simulink model "Sim_Multi"  (R2016b)
settings: Solver=ode3  StartTime=0.0  StopTime=sim_time  FixedStep=t_sim  MaxStep=t_control  RelTol=1e-5  EnableMultiTasking=on
values from neighbouring files (symbols this model uses):
  Att_init = [0;0;0] * d2r    [Init_Multi.m]
  Blade_flapping = 0    [Init_Multi.m]
  C_D = 0.40    (= 0.4)    [Init_Multi.m]
  CoG_nominal = [0;0;0.001]    [Init_Multi.m]
  CoG_real = [0;0;0.001]    [Init_Multi.m]
  Coriolis_correction = 1    [Init_Multi.m]
  d2r = pi/180    (= 0.0174532925199)    [Init_Multi.m]
  Dyn_thrust = 0    [Init_Multi.m]
  g = 9.80665    [Init_Multi.m]
  J_nominal = [Jxx Jxy Jxz;Jyx Jyy Jyz;Jzx Jzy Jzz]    [Init_Multi.m]
  J_real = [Jxx Jxy Jxz;Jyx Jyy Jyz;Jzx Jzy Jzz]    [Init_Multi.m]
  k1 = -1.125    [Init_Multi.m]
  k2 = -1.372    [Init_Multi.m]
  k3 = -1.718    [Init_Multi.m]
  k4 = -0.655    [Init_Multi.m]
  k_a1s = 1.5 / 4.0    (= 0.375)    [Init_Multi.m]
  k_beta = 0.23    [Init_Multi.m]
  kappa = 1.00    (= 1)    [Init_Multi.m]
  Kff_1 = 0.7*[1;1;0.95]    [Init_Multi.m]
  Ki_1 = 10*[1;1;1.5]    [Init_Multi.m]
  Kp_1 = 15*[1;1;1.5]    [Init_Multi.m]
  mass_nominal = 0.550    (= 0.55)    [Init_Multi.m]
  mass_real = 0.550    (= 0.55)    [Init_Multi.m]
  max_thrust = max_thrust + (MotorMatrix_nominal(i,7)*MotorMatrix_nominal(i,12)+MotorMatrix_nominal(i,8)*MotorMatrix_nominal(i,12)^2)    [Init_Multi.m]
  MaxRate_cmd = [360;360;120] * d2r    [Init_Multi.m]
  min_thrust = min_thrust + (MotorMatrix_nominal(i,7)*MotorMatrix_nominal(i,11)+MotorMatrix_nominal(i,8)*MotorMatrix_nominal(i,11)^2)    [Init_Multi.m]
  MotorMap = B' * inv(B * B')    [Init_Multi.m]
  MotorMatrix_nominal = [045 , 0.170 , -0.028 , -1 , 1.0 , 0.010 , [9.6820 , 0.010872]*1e-5 , [1.4504 , 0.0016312]*1e-6 , 0000 , 6000 , [0.0 , 0.0 , 0.0] , 8*2.54/100 , 11/1000;                         135 , 0.170 , -0.028 , +1 , 1.0 , 0.010 , [9.6820 , 0.010872]*1e-5 , [1.4504 , 0.0016312]*1e-6 , 0000 , 6000 , [0.0 , 0.0 , 0.0] , 8*2.54/100 , 11/1000;                         225 , 0.170 , -0.028 , -1 , 1.0 , 0.010 , [9. ...(+284 chars)    [Init_Multi.m]
  MotorMatrix_real = [045 , 0.170 , -0.028 , -1 , 1.0 , 0.010 , [9.6820 , 0.010872]*1e-5 , [1.4504 , 0.0016312]*1e-6 , 0000 , 6000 , [0.0 , 0.0 , 0.0] , 8*2.54/100 , 11/1000;                      135 , 0.170 , -0.028 , +1 , 1.0 , 0.010 , [9.6820 , 0.010872]*1e-5 , [1.4504 , 0.0016312]*1e-6 , 0000 , 6000 , [0.0 , 0.0 , 0.0] , 8*2.54/100 , 11/1000;                      225 , 0.170 , -0.028 , -1 , 1.0 , 0.010 , [9.6820 , ...(+275 chars)    [Init_Multi.m]
  Noise_flag = 0    [Init_Multi.m]
  omega_init = [0;0;0]    [Init_Multi.m]
  q_init = rpy2quat(Att_init)    [Init_Multi.m]
  r2d = 180/pi    (= 57.2957795131)    [Init_Multi.m]
  rho = 1.225    [Init_Multi.m]
  rpm2radpersec = 2*pi/60    (= 0.10471975512)    [Init_Multi.m]
  rpm_init = 3104.5025852    [Init_Multi.m]
  Surface_params = [a;b;c]    [Init_Multi.m]
  t_control = 1/500    (= 0.002)    [Init_Multi.m]
  t_sim = t_control/2    (= 0.001)    [Init_Multi.m]
  thrust_gain = (max_thrust - min_thrust) / 1000    (= 0)    [Init_Multi.m]
  thrust_offset = min_thrust    (= 0)    [Init_Multi.m]
  thrust_reserve = 0.10    (= 0.1)    [Init_Multi.m]
  v_h = 4.0    (= 4)    [Init_Multi.m]
  Vb_init = [0;0;0]    [Init_Multi.m]
  Vi_init = R_IB_init' * Vb_init    [Init_Multi.m]
  Xi_init = [0;0;0]    [Init_Multi.m]
undefined symbols (not defined in the file or in its folder): DiscIntNeverNeededParam, rpy2quat, thrust2rpm
libraries: simulink x17
(part 4 of 4)

== system Sim_Multi/True dynamic system representation of a multirotor UAV/Force//Moment computation/Forces and moments generated by spinning propellers/For Each Subsystem/Thrust//moment vector for each propeller (Body axes)/Compute dynamic motor thrust and moments/Dynamic thrust ratio/Angle of attack and airspeed magnitude/Nonzero airspeed ==
  Airspeed (Motor) : Inport
  Action Port : ActionPort  ActionType=else
  Demux : Demux  Outputs=[2,1]
  Divide1 : Product  Inputs=/*
  Trigonometric Function : Trigonometry  Operator=atan
  norm1 : Subsystem
  AoA (rad) : Outport
  wires:
  Trigonometric Function/1 -> AoA (rad)/1
  Demux/1 -> norm1/1(u)  "Airspeed xy component"
  Demux/2 -> Divide1/2  "Airspeed z component"
  norm1/1(||u||) -> Divide1/1
  Divide1/1 -> Trigonometric Function/1
  Airspeed (Motor)/1 -> Demux/1

== system Sim_Multi/True dynamic system representation of a multirotor UAV/Force//Moment computation/Forces and moments generated by spinning propellers/For Each Subsystem/Thrust//moment vector for each propeller (Body axes)/Compute dynamic motor thrust and moments/Dynamic thrust ratio/Angle of attack and airspeed magnitude/Zero airspeed ==
  Airspeed (Motor) : Inport
  Action Port : ActionPort  ActionType=then
  Constant : Constant  Value=0
  Terminator : Terminator
  AoA (rad) : Outport  InitialOutput=[0]
  wires:
  Airspeed (Motor)/1 -> Terminator/1  "Airspeed (Motor axes)"
  Constant/1 -> AoA (rad)/1

== system Sim_Multi/True dynamic system representation of a multirotor UAV/Force//Moment computation/Forces and moments generated by spinning propellers/For Each Subsystem/Thrust//moment vector for each propeller (Body axes)/Compute dynamic motor thrust and moments/Dynamic thrust ratio/Angle of attack and airspeed magnitude/norm2 ==
  u : Inport
  Complex to Real-Imag : ComplexToRealImag  Output=Real
  Sqrt : Sqrt  SaturateOnIntegerOverflow=on
  dot_product : Subsystem
  ||u|| : Outport
  wires:
  u/1 -> dot_product/1(u), dot_product/2(v)
  dot_product/1(u.v) -> Sqrt/1
  Sqrt/1 -> Complex to Real-Imag/1
  Complex to Real-Imag/1 -> ||u||/1

== system Sim_Multi/True dynamic system representation of a multirotor UAV/Force//Moment computation/Forces and moments generated by spinning propellers/For Each Subsystem/Thrust//moment vector for each propeller (Body axes)/Compute dynamic motor thrust and moments/Dynamic thrust ratio/Flight modes of the propeller/Normal working state vc//vh >= 0 ==
  v_c : Inport
  Action Port : ActionPort  ActionType=then
  Gain : Gain  Gain=0.5
  Induced velocity at hover : Constant  Value=v_h
  Product : Product
  Product1 : Product
  Sqrt : Sqrt  SaturateOnIntegerOverflow=on
  Sum : Sum  Inputs=|-+
  Sum1 : Sum  Inputs=|++
  v_i : Outport
  wires:
  v_c/1 -> Gain/1  "Climb velocity"
  Gain/1 -> Product/2, Product/1, Sum/1
  Sqrt/1 -> Sum/2
  Sum/1 -> v_i/1
  Product/1 -> Sum1/1
  Sum1/1 -> Sqrt/1
  Induced velocity at hover/1 -> Product1/2, Product1/1
  Product1/1 -> Sum1/2

== system Sim_Multi/True dynamic system representation of a multirotor UAV/Force//Moment computation/Forces and moments generated by spinning propellers/For Each Subsystem/Thrust//moment vector for each propeller (Body axes)/Compute dynamic motor thrust and moments/Dynamic thrust ratio/Flight modes of the propeller/Vortex ring state -2 <= vc//vh < 0  ==
  v_c : Inport
  Action Port : ActionPort  ActionType=elseif
  Add : Sum  Inputs=+++++
  Constant : Constant  Value=kappa
  Divide : Product  Inputs=*/
  Gain : Gain  Gain=k1
  Gain1 : Gain  Gain=k2
  Gain2 : Gain  Gain=k3
  Gain3 : Gain  Gain=k4
  Induced velocity at hover : Constant  Value=v_h
  Product{,1..3} (4 alike) : Product
  v_i : Outport
  wires:
  v_c/1 -> Divide/1  "Climb velocity"
  Induced velocity at hover/1 -> Product3/2, Divide/2
  Divide/1 -> Product2/2, Product1/2, Product/2, Product/1, Gain/1
  Product/1 -> Gain1/1, Product1/1
  Product1/1 -> Gain2/1, Product2/1
  Product2/1 -> Gain3/1
  Gain3/1 -> Add/5
  Gain2/1 -> Add/4
  Gain1/1 -> Add/3
  Gain/1 -> Add/2
  Constant/1 -> Add/1
  Add/1 -> Product3/1
  Product3/1 -> v_i/1

== system Sim_Multi/True dynamic system representation of a multirotor UAV/Force//Moment computation/Forces and moments generated by spinning propellers/For Each Subsystem/Thrust//moment vector for each propeller (Body axes)/Compute dynamic motor thrust and moments/Dynamic thrust ratio/Flight modes of the propeller/Windmill braking state vc//vh < -2 ==
  v_c : Inport
  Action Port : ActionPort  ActionType=else
  Gain : Gain  Gain=0.5
  Induced velocity at hover : Constant  Value=v_h
  Product : Product
  Product1 : Product
  Sqrt : Sqrt  SaturateOnIntegerOverflow=on
  Sum : Sum  Inputs=|--
  Sum1 : Sum  Inputs=|+-
  v_i : Outport
  wires:
  v_c/1 -> Gain/1  "Climb velocity"
  Gain/1 -> Product/2, Product/1, Sum/1
  Sqrt/1 -> Sum/2
  Sum/1 -> v_i/1
  Product/1 -> Sum1/1
  Sum1/1 -> Sqrt/1
  Induced velocity at hover/1 -> Product1/2, Product1/1
  Product1/1 -> Sum1/2

== system Sim_Multi/True dynamic system representation of a multirotor UAV/Force//Moment computation/Forces and moments generated by spinning propellers/For Each Subsystem/Thrust//moment vector for each propeller (Body axes)/Compute dynamic motor thrust and moments/Gyroscopic torque/Cross Product/Subsystem ==
  u : Inport
  v : Inport  Port=2
  Demux : Demux  Outputs=3
  Demux1 : Demux  Outputs=3
  Mux : Mux  Inputs=3
  Product : Product
  Product1 : Product
  Product2 : Product
  Positive elements : Outport
  wires:
  Mux/1 -> Positive elements/1
  v/1 -> Demux1/1
  u/1 -> Demux/1
  Demux/2 -> Product/1
  Demux1/3 -> Product/2
  Demux/3 -> Product1/1
  Demux1/1 -> Product1/2
  Demux/1 -> Product2/1
  Demux1/2 -> Product2/2
  Product/1 -> Mux/1
  Product1/1 -> Mux/2
  Product2/1 -> Mux/3

== system Sim_Multi/True dynamic system representation of a multirotor UAV/Force//Moment computation/Forces and moments generated by spinning propellers/For Each Subsystem/Thrust//moment vector for each propeller (Body axes)/Compute dynamic motor thrust and moments/Gyroscopic torque/Cross Product/Subsystem1 ==
  u : Inport
  v : Inport  Port=2
  Demux : Demux  Outputs=3
  Demux1 : Demux  Outputs=3
  Mux : Mux  Inputs=3
  Product : Product
  Product1 : Product
  Product2 : Product
  Negative elements : Outport
  wires:
  Mux/1 -> Negative elements/1
  v/1 -> Demux1/1
  u/1 -> Demux/1
  Product/1 -> Mux/1
  Product1/1 -> Mux/2
  Product2/1 -> Mux/3
  Demux/3 -> Product/1
  Demux1/2 -> Product/2
  Demux/1 -> Product1/1
  Demux1/3 -> Product1/2
  Demux/2 -> Product2/1
  Demux1/1 -> Product2/2

== system Sim_Multi/True dynamic system representation of a multirotor UAV/Force//Moment computation/Forces and moments generated by spinning propellers/For Each Subsystem/Thrust//moment vector for each propeller (Body axes)/Compute dynamic motor thrust and moments/Blade flapping computations/Nonzero airspeed in rotor plane/norm/dot_product ==
  u : Inport
  v : Inport  Port=2
  Product : Product  Multiplication=Matrix(*)  RndMeth=Zero
  Reshape : Reshape  OutputDimensionality=Column vector (2-D)
  Reshape1 : Reshape  OutputDimensionality=Column vector (2-D)
  transpose : Math  Operator=transpose  SaturateOnIntegerOverflow=on
  u.v : Outport
  wires:
  v/1 -> Reshape1/1
  u/1 -> Reshape/1
  Reshape/1 -> transpose/1
  transpose/1 -> Product/1
  Reshape1/1 -> Product/2
  Product/1 -> u.v/1

== system Sim_Multi/True dynamic system representation of a multirotor UAV/Force//Moment computation/Forces and moments generated by spinning propellers/For Each Subsystem/Thrust//moment vector for each propeller (Body axes)/Compute dynamic motor thrust and moments/Dynamic thrust ratio/Angle of attack and airspeed magnitude/Nonzero airspeed/norm1 ==
  u : Inport
  Complex to Real-Imag : ComplexToRealImag  Output=Real
  Sqrt : Sqrt  SaturateOnIntegerOverflow=on
  dot_product : Subsystem
  ||u|| : Outport
  wires:
  u/1 -> dot_product/1(u), dot_product/2(v)
  dot_product/1(u.v) -> Sqrt/1
  Sqrt/1 -> Complex to Real-Imag/1
  Complex to Real-Imag/1 -> ||u||/1

== system Sim_Multi/True dynamic system representation of a multirotor UAV/Force//Moment computation/Forces and moments generated by spinning propellers/For Each Subsystem/Thrust//moment vector for each propeller (Body axes)/Compute dynamic motor thrust and moments/Dynamic thrust ratio/Angle of attack and airspeed magnitude/norm2/dot_product ==
  u : Inport
  v : Inport  Port=2
  Product : Product  Multiplication=Matrix(*)  RndMeth=Zero
  Reshape : Reshape  OutputDimensionality=Column vector (2-D)
  Reshape1 : Reshape  OutputDimensionality=Column vector (2-D)
  transpose : Math  Operator=transpose  SaturateOnIntegerOverflow=on
  u.v : Outport
  wires:
  v/1 -> Reshape1/1
  u/1 -> Reshape/1
  Reshape/1 -> transpose/1
  transpose/1 -> Product/1
  Reshape1/1 -> Product/2
  Product/1 -> u.v/1

== system Sim_Multi/True dynamic system representation of a multirotor UAV/Force//Moment computation/Forces and moments generated by spinning propellers/For Each Subsystem/Thrust//moment vector for each propeller (Body axes)/Compute dynamic motor thrust and moments/Dynamic thrust ratio/Angle of attack and airspeed magnitude/Nonzero airspeed/norm1/dot_product ==
  u : Inport
  v : Inport  Port=2
  Product : Product  Multiplication=Matrix(*)  RndMeth=Zero
  Reshape : Reshape  OutputDimensionality=Column vector (2-D)
  Reshape1 : Reshape  OutputDimensionality=Column vector (2-D)
  transpose : Math  Operator=transpose  SaturateOnIntegerOverflow=on
  u.v : Outport
  wires:
  v/1 -> Reshape1/1
  u/1 -> Reshape/1
  Reshape/1 -> transpose/1
  transpose/1 -> Product/1
  Reshape1/1 -> Product/2
  Product/1 -> u.v/1
